simulink model "Lab3FigureEightDrive"  (R2024a)
settings: Solver=FixedStepDiscrete  StartTime=0.0  StopTime=90  FixedStep=0.01  RelTol=1e-3
undefined symbols (not defined in the file): DiscIntNeverNeededParam
libraries: mobileRoboticsTrainingLib x1
settings Model: PacingRate=5  Creator=Beast  LastModifiedBy=Beast

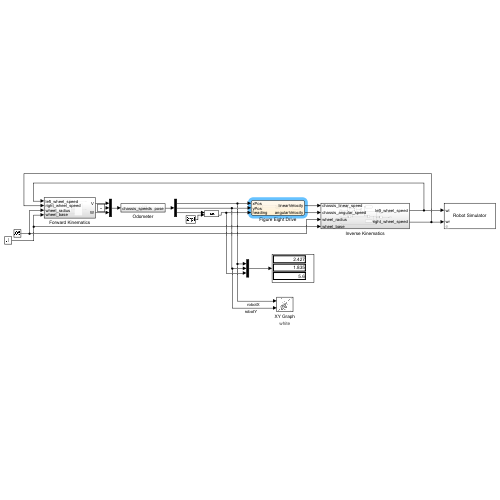
[thumbnail: Simulink's stored preview of the top-level diagram]
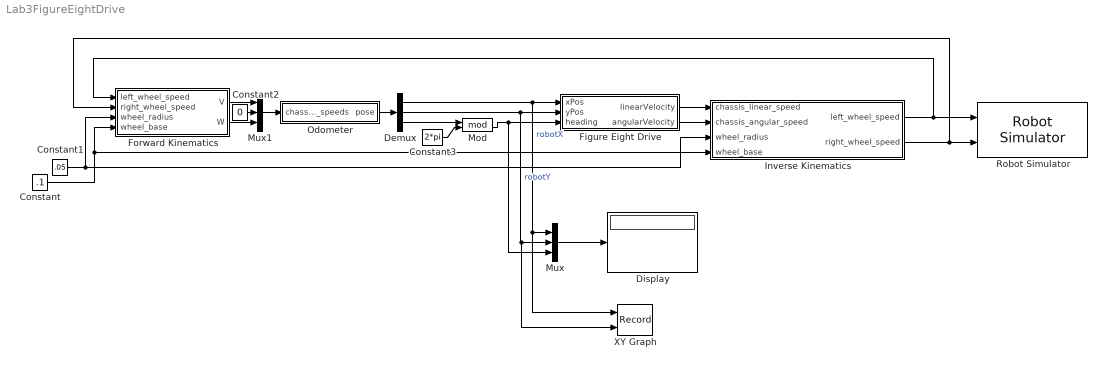
== system Lab3FigureEightDrive ==
  Constant : Constant  Value=.1
  Constant1 : Constant  Value=.05
  Constant2 : Constant  Value=0
  Constant3 : Constant  Value=2*pi
  Demux : Demux  Outputs=3
  Display : Display
  Figure Eight Drive : Stateflow chart  TreatAsAtomicUnit=on
  Forward Kinematics : Subsystem
  Inverse Kinematics : Subsystem
  Mod : Math  Operator=mod
  Mux : Mux  Inputs=3
  Mux1 : Mux  Inputs=3
  Odometer : Subsystem
  Robot Simulator : mobileRoboticsTrainingLib/Robot Simulator  Priority=99  mapVar=[]  startX=2  startY=2  startTheta=0  axleLength=0.1  wheelR=0.05
  XY Graph : Record  FileSettingsInternal="{\"entries\":[{\"content\":{\"excelSettings\":{\"content\":{},\"type\":\"Streamout.ExcelSettings\"}},\"type\":\"Streamout.FileSettingStorage\",\"uuid\":\"\"}],\"packageUris\":[\"http:\\/\\/schema.mathworks.com\\/mf0\\/streamout_blocks\\/R2020a\"],\"version\":\"1.0\"}"  Layout=[1 1]  SignalsInternal="{\"entries\":[{\"content\":{\"signals\":[{\"content\":{\"blockPath\":[],\"dimensions\":[1],\"domain\":\"\",\"lineColor\":\"#a2142f\",\"plots\":[ 1 ],\"port\":1,\"sid\":[\"\"],\"signalID\":1,\"signalName\":\"robotX\"},\"type\":\"RecordBlkView.Signal\",\"uuid\":\"\"},{\"content\":{\"blockPath\":[],\"dimensions\":[1],\"domain\":\"\",\"lineColor\":\"#139fff\",\"plots\":[ 1 ],\"port\":2,\"sid\":[\"\"],\"signalID\":2,\"signalName\":\"robotY\"},\"type\":\"RecordBlkView.Signal\",\"uuid\":\"\"}]},\"type\":\"RecordBlkView.InputSignals\",\"uuid\":\"\"}],\"packageUris\":[\"http:\\/\\/schema.mathworks.com\\/mf0\\/streamout_blocks\\/R2020a\"],\"version\":\"1.0\"}"  VisualizationBindings="{\"xyplotplugin\":{\"info\":[{\"series\":[{\"bindingParametersList\":[{\"parameter\":\"X-Axis\",\"signalID\":1,\"signalName\":\"robotX\"},{\"parameter\":\"Y-Axis\",\"signalID\":2,\"signalName\":\"robotY\"}],\"seriesID\":0}],\"subplotID\":1}]}}"  CompatibilityTag=XY
      settings: AttributesFormatString=%<BackgroundColor>
  wires:
  Inverse Kinematics/1(left_wheel_speed) -> Forward Kinematics/1(left_wheel_speed), Robot Simulator/1
  Forward Kinematics/1(V) -> Mux1/1
  Inverse Kinematics/2(right_wheel_speed) -> Robot Simulator/2, Forward Kinematics/2(right_wheel_speed)
  Mux1/1 -> Odometer/1(chassis_speeds)
  Mod/1 -> Mux/3, Figure Eight Drive/3(heading)
  Constant3/1 -> Mod/2
  Constant2/1 -> Mux1/2
  Demux/2 -> XY Graph/2, Mux/2, Figure Eight Drive/2(yPos)  "robotY"
  Odometer/1(pose) -> Demux/1
  Forward Kinematics/2(W) -> Mux1/3
  Mux/1 -> Display/1
  Demux/3 -> Mod/1
  Constant1/1 -> Forward Kinematics/3(wheel_radius), Inverse Kinematics/3(wheel_radius)
  Figure Eight Drive/2(angularVelocity) -> Inverse Kinematics/2(chassis_angular_speed)
  Demux/1 -> XY Graph/1, Mux/1, Figure Eight Drive/1(xPos)  "robotX"
  Constant/1 -> Forward Kinematics/4(wheel_base), Inverse Kinematics/4(wheel_base)
  Figure Eight Drive/1(linearVelocity) -> Inverse Kinematics/1(chassis_linear_speed)

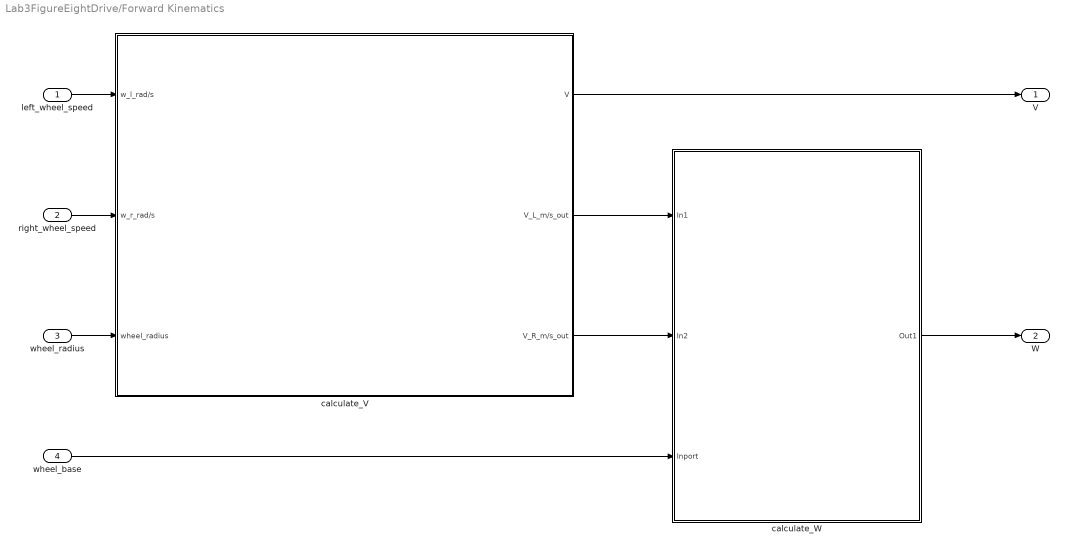
== system Lab3FigureEightDrive/Forward Kinematics ==
  left_wheel_speed : Inport
  right_wheel_speed : Inport  Port=2
  wheel_radius : Inport  Port=3
  wheel_base : Inport  Port=4
  calculate_V : Subsystem
  calculate_W : Subsystem
  V : Outport
  W : Outport  Port=2
  wires:
  calculate_V/1(V) -> V/1
  right_wheel_speed/1 -> calculate_V/2(w_r_rad/s)
  left_wheel_speed/1 -> calculate_V/1(w_l_rad/s)
  calculate_V/2(V_L_m/s_out) -> calculate_W/1(In1)
  calculate_W/1(Out1) -> W/1
  calculate_V/3(V_R_m/s_out) -> calculate_W/2(In2)
  wheel_radius/1 -> calculate_V/3(wheel_radius)
  wheel_base/1 -> calculate_W/3(Inport)

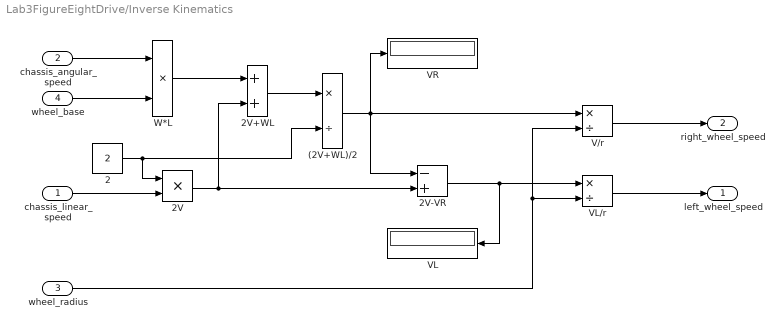
== system Lab3FigureEightDrive/Inverse Kinematics ==
  chassis_linear_speed : Inport
  chassis_angular_speed : Inport  Port=2
  wheel_radius : Inport  Port=3
  wheel_base : Inport  Port=4
  (2V+WL)/2 : Product  Inputs=*/
  2 : Constant  Value=2
  2V : Product
  2V+WL : Sum
  2V-VR : Sum  Inputs=-+
  V/r : Product  Inputs=*/
  VL : Display
  VL/r : Product  Inputs=*/
  VR : Display
  W*L : Product
  left_wheel_speed : Outport
  right_wheel_speed : Outport  Port=2
  wires:
  2/1 -> 2V/1, (2V+WL)/2/2
  W*L/1 -> 2V+WL/1
  (2V+WL)/2/1 -> 2V-VR/1, V/r/1, VR/1
  wheel_radius/1 -> V/r/2, VL/r/2
  2V-VR/1 -> VL/r/1, VL/1
  2V/1 -> 2V+WL/2, 2V-VR/2
  VL/r/1 -> left_wheel_speed/1
  2V+WL/1 -> (2V+WL)/2/1
  V/r/1 -> right_wheel_speed/1
  chassis_linear_speed/1 -> 2V/2
  chassis_angular_speed/1 -> W*L/1
  wheel_base/1 -> W*L/2

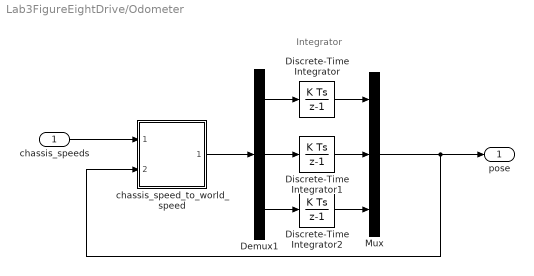
== system Lab3FigureEightDrive/Odometer ==
  note: Integrator
  chassis_speeds : Inport
  Demux1 : Demux  Outputs=3
  Discrete-Time Integrator : DiscreteIntegrator  InitialCondition=2  SampleTime=-1  ICPrevOutput=DiscIntNeverNeededParam  ICPrevScaledInput=DiscIntNeverNeededParam
  Discrete-Time Integrator1 : DiscreteIntegrator  InitialCondition=2  SampleTime=-1  ICPrevOutput=DiscIntNeverNeededParam  ICPrevScaledInput=DiscIntNeverNeededParam
  Discrete-Time Integrator2 : DiscreteIntegrator  SampleTime=-1  ICPrevOutput=DiscIntNeverNeededParam  ICPrevScaledInput=DiscIntNeverNeededParam
  Mux : Mux  Inputs=3
  chassis_speed_to_world_speed : Subsystem
  pose : Outport  VectorParamsAs1DForOutWhenUnconnected=off
  wires:
  Discrete-Time Integrator/1 -> Mux/1
  Demux1/2 -> Discrete-Time Integrator1/1
  Discrete-Time Integrator2/1 -> Mux/3
  Mux/1 -> chassis_speed_to_world_speed/2(last_pose), pose/1
  Demux1/3 -> Discrete-Time Integrator2/1
  Discrete-Time Integrator1/1 -> Mux/2
  Demux1/1 -> Discrete-Time Integrator/1
  chassis_speed_to_world_speed/1(global_velocity) -> Demux1/1
  chassis_speeds/1 -> chassis_speed_to_world_speed/1(robot_velocity)

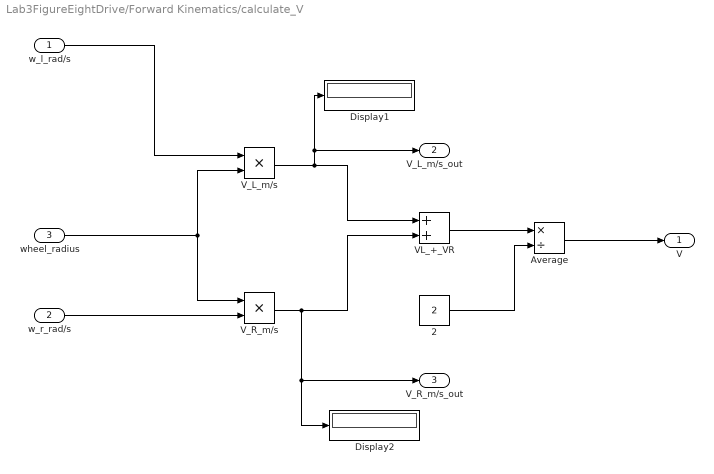
== system Lab3FigureEightDrive/Forward Kinematics/calculate_V ==
  w_l_rad/s : Inport
  w_r_rad/s : Inport  Port=2
  wheel_radius : Inport  Port=3
  2 : Constant  Value=2
  Average : Product  Inputs=*/
  Display1 : Display
  Display2 : Display
  VL_+_VR : Sum
  V_L_m/s : Product
  V_R_m/s : Product
  V : Outport
  V_L_m/s_out : Outport  Port=2
  V_R_m/s_out : Outport  Port=3
  wires:
  w_r_rad/s/1 -> V_R_m/s/2
  VL_+_VR/1 -> Average/1
  wheel_radius/1 -> V_L_m/s/2, V_R_m/s/1
  V_L_m/s/1 -> Display1/1, V_L_m/s_out/1, VL_+_VR/1
  V_R_m/s/1 -> V_R_m/s_out/1, Display2/1, VL_+_VR/2
  2/1 -> Average/2
  w_l_rad/s/1 -> V_L_m/s/1
  Average/1 -> V/1

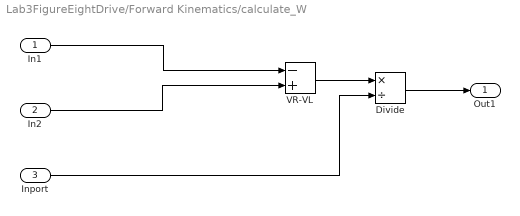
== system Lab3FigureEightDrive/Forward Kinematics/calculate_W ==
  In1 : Inport
  In2 : Inport  Port=2
  Inport : Inport  Port=3
  Divide : Product  Inputs=*/
  VR-VL : Sum  Inputs=-+
  Out1 : Outport
  wires:
  Inport/1 -> Divide/2
  VR-VL/1 -> Divide/1
  In2/1 -> VR-VL/2
  In1/1 -> VR-VL/1
  Divide/1 -> Out1/1

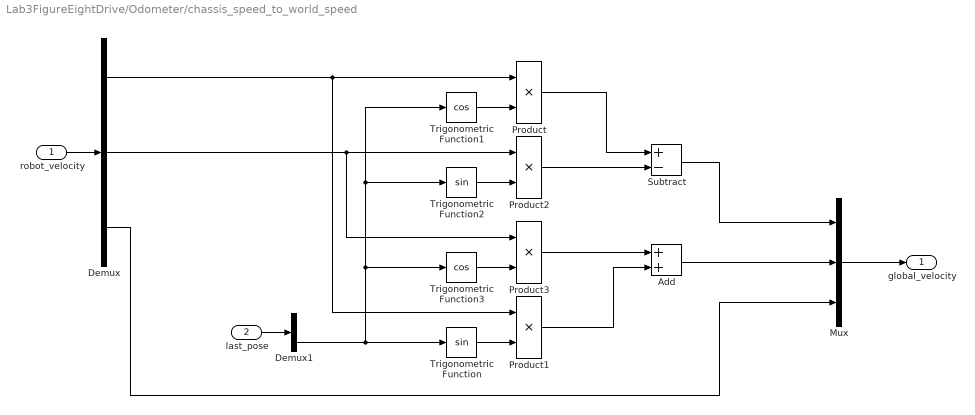
== system Lab3FigureEightDrive/Odometer/chassis_speed_to_world_speed ==
  robot_velocity : Inport
  last_pose : Inport  Port=2
  Add : Sum
  Demux : Demux  Outputs=3
  Demux1 : Demux  Outputs=3
  Mux : Mux  Inputs=3
  Product{,1..3} (4 alike) : Product
  Subtract : Sum  Inputs=+-
  Trigonometric Function : Trigonometry
  Trigonometric Function1 : Trigonometry  Operator=cos
  Trigonometric Function2 : Trigonometry
  Trigonometric Function3 : Trigonometry  Operator=cos
  global_velocity : Outport  VectorParamsAs1DForOutWhenUnconnected=off
  wires:
  Demux1/3 -> Trigonometric Function1/1, Trigonometric Function2/1, Trigonometric Function3/1, Trigonometric Function/1
  Trigonometric Function3/1 -> Product3/2
  Trigonometric Function/1 -> Product1/2
  robot_velocity/1 -> Demux/1
  Product1/1 -> Add/2
  Product2/1 -> Subtract/2
  Product/1 -> Subtract/1
  Demux/3 -> Mux/3
  Add/1 -> Mux/2
  Trigonometric Function1/1 -> Product/2
  Subtract/1 -> Mux/1
  Demux/1 -> Product/1, Product1/1
  Product3/1 -> Add/1
  Demux/2 -> Product3/1, Product2/1
  Mux/1 -> global_velocity/1
  Trigonometric Function2/1 -> Product2/2
  last_pose/1 -> Demux1/1

== stateflow chart Lab3FigureEightDrive/Figure Eight Drive ==
  state CircleDriveLeft
    entry:
    angularVelocity = 1.33333;
    targetX = xPos;
    targetY = yPos;
  state Intermediate1
  state CircleDriveRight
    entry:
    angularVelocity = -1.33333;
    targetX = xPos;
    targetY = yPos;
  state Intermediate2
  note: These states ensure that we have left the starting position
  (default) -> CircleDriveLeft
  CircleDriveLeft -> Intermediate1 : [abs(targetX - xPos) > .01 && abs(targetY - yPos) > .01]
  Intermediate1 -> CircleDriveRight : [abs(targetX - xPos) < .01 && abs(targetY - yPos) < .01]
  Intermediate2 -> CircleDriveLeft : [abs(targetX - xPos) < .01 && abs(targetY - yPos) < .01]
  CircleDriveRight -> Intermediate2 : [abs(targetX - xPos) > .01 && abs(targetY - yPos) > .01]
  data: xPos input; yPos input; linearVelocity output =1; heading input; angularVelocity output; targetX local; targetY local; targetHeading local
